simulink model "slexMFSKMultiTargetsExample"  (R2019a)
settings: Solver=FixedStepDiscrete  StartTime=0.0  StopTime=paramMFSKMT.T  RelTol=1e-3  EnableMultiTasking=on
PreLoadFcn:
  | helperslexMFSKMultiTargetsParam
undefined symbols (not defined in the file or in its folder): paramMFSKMT
libraries: phasedenvlib x7, phasedtxrxlib x2, phaseddetectlib x2, dspxfrm3 x2, phasedwavlib x1, dspsolvers x1
CloseFcn:
  | clear paramMFSKMT
Description:
  | FMCW Radar Range Estimation
  | 
  | This model shows how to use a FMCW radar to estimate a target's range.
settings Model: Creator=The MathWorks, Inc.  LastModifiedBy=The MathWorks, Inc.
settings DataIOCC: LimitDataPoints=on  SaveFormat=Array  ReturnWorkspaceOutputs=off
settings OptimizationCC: LifeSpan=inf
settings DebuggingCC: ReadBeforeWriteMsg=DisableAll  WriteAfterWriteMsg=DisableAll  WriteAfterReadMsg=DisableAll  UnderspecifiedInitializationDetection=Classic  MergeDetectMultiDrivingBlocksExec=none  SolverPrmCheckMsg=warning  MultiTaskDSMMsg=none  PregeneratedLibrarySubsystemCodeDiagnostic=none  SFUnexpectedBacktrackingDiag=warning  SFNoUnconditionalDefaultTransitionDiag=warning  SFExecutionAtInitializationDiag=none  ArithmeticOperatorsInVariantConditions=warning
settings HardwareCC: ProdBitPerPointer=32  ProdBitPerSizeT=32  ProdBitPerPtrDiffT=32  ProdLargestAtomicFloat=None  ProdIntDivRoundTo=Undefined  ProdEndianess=Unspecified  ProdWordSize=32  ProdHWDeviceType=32-bit Generic
settings ModelReferenceCC: UpdateModelReferenceTargets=IfOutOfDate  PropagateSignalLabelsOutOfModel=off
settings SFSimCC: SFSimEcho=off  SimUseLocalCustomCode=off
settings RTWCC: RTWUseLocalCustomCode=off
settings CodeAppCC: StateflowObjectComments=on
settings GRTTargetCC: TargetLangStandard=C89/C90 (ANSI)  GeneratePreprocessorConditionals=Disable all
settings ConfigComp: CovMetricSettings=dw  CovHtmlReporting=on  CovSaveCumulativeToWorkspaceVar=on  CovSaveSingleToWorkspaceVar=on  CovExternalEMLEnable=off  CovSFcnEnable=off

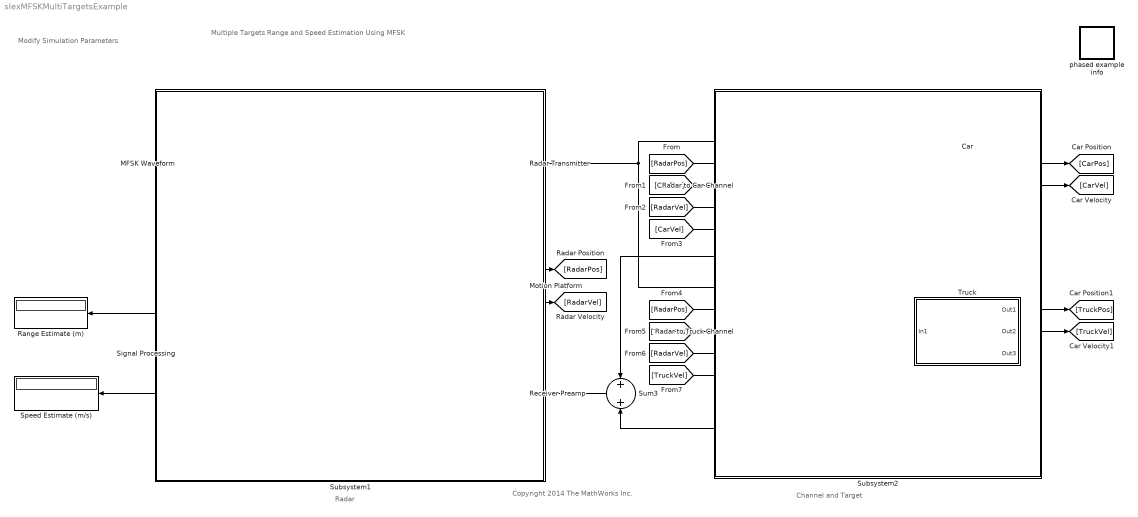
== system slexMFSKMultiTargetsExample ==
  note: Copyright 2014 The MathWorks Inc.
  note: Radar
  note: Channel and Target
  note: Multiple Targets Range and Speed Estimation Using MFSK
  note: Modify Simulation Parameters
  Car : Subsystem
      mask Display:
      | disp('Car')
      | port_label('output',1,'Pos')
      | port_label('output',2,'Vel')
      | port_label('output',3,'Sig')
  MFSK Waveform : phasedwavlib/MFSK Waveform  SampleRate=paramMFSKMT.Fs  SweepBandwidth=paramMFSKMT.bw  StepTime=paramMFSKMT.Tstep  StepsPerSweep=paramMFSKMT.Nstep  FrequencyOffset=paramMFSKMT.Foffset  OutputFormat=Sweeps  NumSamples=100  NumSteps=1  NumSweeps=1  SimulateUsing=Interpreted execution
      settings: SourceProductName=Phased Array System Toolbox  SourceProductBaseCode=AR
  Motion Platform : phasedenvlib/Motion Platform  MotionModel=Velocity  InitialPosition=paramMFSKMT.RadarPos  InitialVelocity=[ 0; 0; 0 ]  VelocitySource=Property  Velocity=paramMFSKMT.RadarVel  AccelerationSource=Property  Acceleration=[0;0;0]  CustomTrajectory=[ 0, 0, 0, 0, 0, 0, 0; 1, 0, 0, 0, 0, 0, 0 ]  ScanMode=None  InitialScanAngle=0  AzimuthSpan=[ -60, 60 ]  AzimuthScanRate=10  InitialOrientationAxes=eye( 3 )  OrientationAxesOutputPort=off  ElapsedTimeSource=Auto  SampleRateFromInputCheckbox=on  SampleRate=1e6  SimulateUsing=Interpreted execution
      settings: SourceProductName=Phased Array System Toolbox  SourceProductBaseCode=AR
  Radar Transmitter : phasedtxrxlib/Transmitter  PeakPower=paramMFSKMT.ppow  Gain=paramMFSKMT.TxGain  LossFactor=0  InUseOutputPort=off  CoherentOnTransmit=on  PhaseNoiseOutputPort=off  SeedSource=Auto  Seed=0  SimulateUsing=Interpreted execution
      settings: SourceProductName=Phased Array System Toolbox  SourceProductBaseCode=AR
  Radar to Car Channel : phasedenvlib/Free Space  PropagationSpeed=paramMFSKMT.C  OperatingFrequency=paramMFSKMT.Fc  TwoWayPropagation=on  SampleRateFromInputCheckbox=on  SampleRate=1e6  MaximumDistanceSource=Property  MaximumDistance=500  MaximumNumInputSamplesSource=Auto  MaximumNumInputSamples=1000  SimulateUsing=Interpreted execution
      settings: SourceProductName=Phased Array System Toolbox  SourceProductBaseCode=AR
  Radar to Truck Channel : phasedenvlib/Free Space  PropagationSpeed=paramMFSKMT.C  OperatingFrequency=paramMFSKMT.Fc  TwoWayPropagation=on  SampleRateFromInputCheckbox=on  SampleRate=1e6  MaximumDistanceSource=Property  MaximumDistance=500  MaximumNumInputSamplesSource=Auto  MaximumNumInputSamples=1000  SimulateUsing=Interpreted execution
      settings: SourceProductName=Phased Array System Toolbox  SourceProductBaseCode=AR
  Range Estimate (m) : Display
  Receiver Preamp : phasedtxrxlib/Receiver Preamp  Gain=paramMFSKMT.RxGain  LossFactor=0  NoiseMethod=Noise temperature  NoiseFigure=paramMFSKMT.NF  ReferenceTemperature=290  SampleRateFromInputCheckbox=on  SampleRate=1e6  NoisePower=0  EnableInputPort=off  PhaseNoiseInputPort=off  SeedSource=Auto  Seed=0  SimulateUsing=Interpreted execution
      settings: SourceProductName=Phased Array System Toolbox  SourceProductBaseCode=AR
  Signal Processing : Subsystem
      mask Display:
      | disp('Signal\nProcessing')
      | port_label('input',1,'Ref')
      | port_label('input',2,'Echo')
      | port_label('output',1,'Range')
      | port_label('output',2,'Speed')
  Speed Estimate (m/s) : Display
  Subsystem1 : Subsystem
  Subsystem2 : Subsystem
  Sum3 : Sum  Inputs=+|+
  Truck : Subsystem
      mask Display:
      | disp('Truck')
      | port_label('output',1,'Pos')
      | port_label('output',2,'Vel')
      | port_label('output',3,'Sig')
  phased example info : Subsystem
      settings: OpenFcn=|
      | modelname = 'slexFMCWExample';
      | helpview(fullfile(matlabroot,'help','phased','helptargets.map'),sprintf('%sExample',modelname));
      | clear modelname;
      mask Display: disp('Info')
  wires:
  MFSK Waveform/1 -> Signal Processing/1(In1), Radar Transmitter/1
  [RadarPos] -> Radar to Car Channel/2
  [CarPos] -> Radar to Car Channel/3
  [RadarVel] -> Radar to Car Channel/4
  [CarVel] -> Radar to Car Channel/5
  Radar Transmitter/1 -> Radar to Truck Channel/1, Radar to Car Channel/1
  Motion Platform/1 -> [RadarPos]
  Motion Platform/2 -> [RadarVel]
  Radar to Car Channel/1 -> Car/1(In1)
  Car/1(Out1) -> [CarPos]
  Car/2(Out2) -> [CarVel]
  Truck/1(Out1) -> [TruckPos]
  Truck/2(Out2) -> [TruckVel]
  Radar to Truck Channel/1 -> Truck/1(In1)
  [RadarPos] -> Radar to Truck Channel/2
  [TruckPos] -> Radar to Truck Channel/3
  [RadarVel] -> Radar to Truck Channel/4
  [TruckVel] -> Radar to Truck Channel/5
  Car/3(Out3) -> Sum3/1
  Sum3/1 -> Receiver Preamp/1
  Truck/3(Out3) -> Sum3/2
  Receiver Preamp/1 -> Signal Processing/2(In2)
  Signal Processing/1(Out1) -> Range Estimate (m)/1
  Signal Processing/2(Out2) -> Speed Estimate (m/s)/1

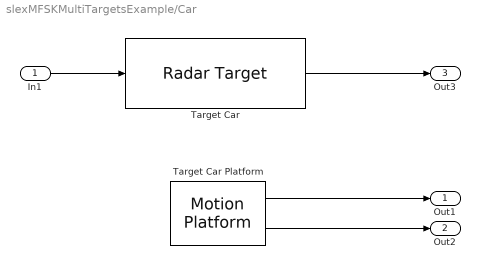
== system slexMFSKMultiTargetsExample/Car ==
  In1 : Inport
  Target Car : phasedenvlib/Radar Target  EnablePolarization=off  Mode=Monostatic  MeanRCSSource=Property  ScatteringMatrixSource=Property  MeanRCS=paramMFSKMT.RCS  ScatteringMatrix=eye( 2 )  Model=Nonfluctuating  PropagationSpeed=paramMFSKMT.C  OperatingFrequency=paramMFSKMT.Fc  SeedSource=Auto  Seed=0  SimulateUsing=Interpreted execution
      settings: SourceProductName=Phased Array System Toolbox  SourceProductBaseCode=AR
  Target Car Platform : phasedenvlib/Motion Platform  MotionModel=Velocity  InitialPosition=paramMFSKMT.CarPos  InitialVelocity=[ 0; 0; 0 ]  VelocitySource=Property  Velocity=paramMFSKMT.CarVel  AccelerationSource=Property  Acceleration=[0;0;0]  CustomTrajectory=[ 0, 0, 0, 0, 0, 0, 0; 1, 0, 0, 0, 0, 0, 0 ]  ScanMode=None  InitialScanAngle=0  AzimuthSpan=[ -60, 60 ]  AzimuthScanRate=10  InitialOrientationAxes=eye( 3 )  OrientationAxesOutputPort=off  ElapsedTimeSource=Auto  SampleRateFromInputCheckbox=on  SampleRate=1e6  SimulateUsing=Interpreted execution
      settings: SourceProductName=Phased Array System Toolbox  SourceProductBaseCode=AR
  Out1 : Outport
  Out2 : Outport  Port=2
  Out3 : Outport  Port=3
  wires:
  Target Car/1 -> Out3/1
  In1/1 -> Target Car/1
  Target Car Platform/1 -> Out1/1
  Target Car Platform/2 -> Out2/1

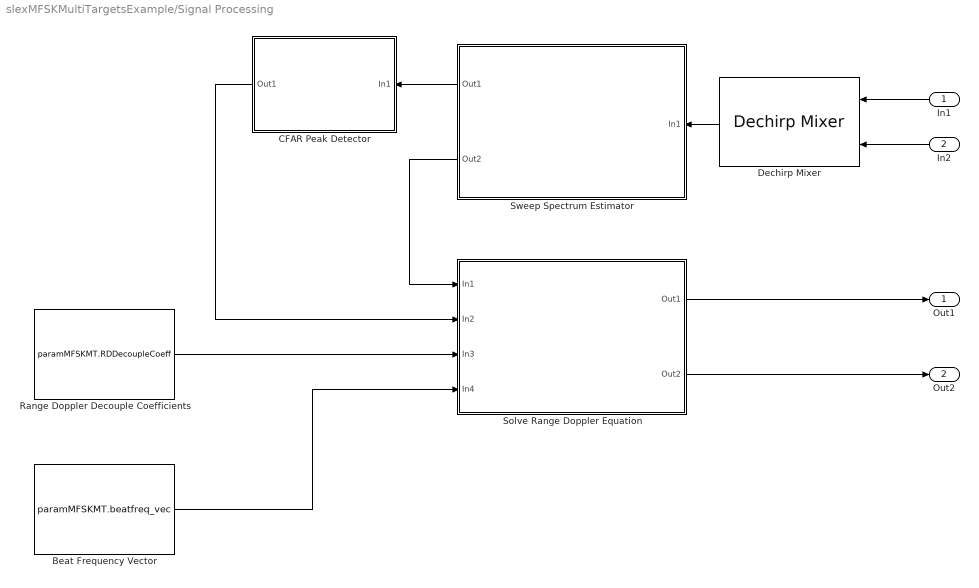
== system slexMFSKMultiTargetsExample/Signal Processing ==
  In1 : Inport
  In2 : Inport  Port=2
  Beat Frequency Vector : Constant  Value=paramMFSKMT.beatfreq_vec  VectorParams1D=off
  CFAR Peak Detector : Subsystem
      mask Display:
      | disp('Peak\nIndex')
      | port_label('output',1,'Idx')
  Dechirp Mixer : phaseddetectlib/Dechirp Mixer
      settings: SourceProductName=Phased Array System Toolbox  SourceProductBaseCode=AR
  Range Doppler Decouple Coefficients : Constant  Value=paramMFSKMT.RDDecoupleCoeff  VectorParams1D=off
  Solve Range Doppler Equation : Subsystem
      mask Display:
      | disp('Range\nDopppler\nSolver\nAX=B')
      | port_label('output',1,'range')
      | port_label('output',2,'speed')
      | port_label('input',2,'Beat Idx')
      | port_label('input',1,'\Delta\Phi_{sweep}','texmode','on')
      | port_label('input',3,'A')
      | port_label('input',4,'freq')
  Sweep Spectrum Estimator : Subsystem
      mask Display:
      | disp('Sweep\nSpectrum')
      | port_label('input',1,'X_d','texmode','on')
      | port_label('output',1,'|F_{sweep}|','texmode','on')
      | port_label('output',2,'\Delta\Phi_{sweep}','texmode','on')
  Out1 : Outport
  Out2 : Outport  Port=2
  wires:
  In2/1 -> Dechirp Mixer/2
  In1/1 -> Dechirp Mixer/1
  Dechirp Mixer/1 -> Sweep Spectrum Estimator/1(In1)
  Sweep Spectrum Estimator/1(Out1) -> CFAR Peak Detector/1(In1)
  Range Doppler Decouple Coefficients/1 -> Solve Range Doppler Equation/3(In3)
  Beat Frequency Vector/1 -> Solve Range Doppler Equation/4(In4)
  Solve Range Doppler Equation/1(Out1) -> Out1/1
  Solve Range Doppler Equation/2(Out2) -> Out2/1
  Sweep Spectrum Estimator/2(Out2) -> Solve Range Doppler Equation/1(In1)
  CFAR Peak Detector/1(Out1) -> Solve Range Doppler Equation/2(In2)

== system slexMFSKMultiTargetsExample/Subsystem1 ==

== system slexMFSKMultiTargetsExample/Subsystem2 ==

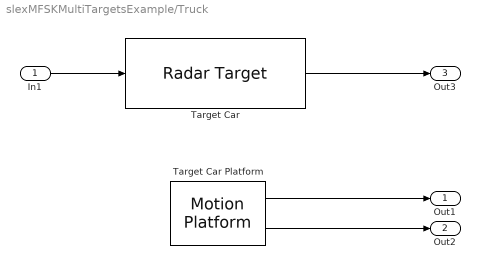
== system slexMFSKMultiTargetsExample/Truck ==
  In1 : Inport
  Target Car : phasedenvlib/Radar Target  EnablePolarization=off  Mode=Monostatic  MeanRCSSource=Property  ScatteringMatrixSource=Property  MeanRCS=paramMFSKMT.TruckRCS  ScatteringMatrix=eye( 2 )  Model=Nonfluctuating  PropagationSpeed=paramMFSKMT.C  OperatingFrequency=paramMFSKMT.Fc  SeedSource=Auto  Seed=0  SimulateUsing=Interpreted execution
      settings: SourceProductName=Phased Array System Toolbox  SourceProductBaseCode=AR
  Target Car Platform : phasedenvlib/Motion Platform  MotionModel=Velocity  InitialPosition=paramMFSKMT.TruckPos  InitialVelocity=[ 0; 0; 0 ]  VelocitySource=Property  Velocity=paramMFSKMT.TruckVel  AccelerationSource=Property  Acceleration=[0;0;0]  CustomTrajectory=[ 0, 0, 0, 0, 0, 0, 0; 1, 0, 0, 0, 0, 0, 0 ]  ScanMode=None  InitialScanAngle=0  AzimuthSpan=[ -60, 60 ]  AzimuthScanRate=10  InitialOrientationAxes=eye( 3 )  OrientationAxesOutputPort=off  ElapsedTimeSource=Auto  SampleRateFromInputCheckbox=on  SampleRate=1e6  SimulateUsing=Interpreted execution
      settings: SourceProductName=Phased Array System Toolbox  SourceProductBaseCode=AR
  Out1 : Outport
  Out2 : Outport  Port=2
  Out3 : Outport  Port=3
  wires:
  Target Car Platform/2 -> Out2/1
  Target Car Platform/1 -> Out1/1
  In1/1 -> Target Car/1
  Target Car/1 -> Out3/1

== system slexMFSKMultiTargetsExample/phased example info ==

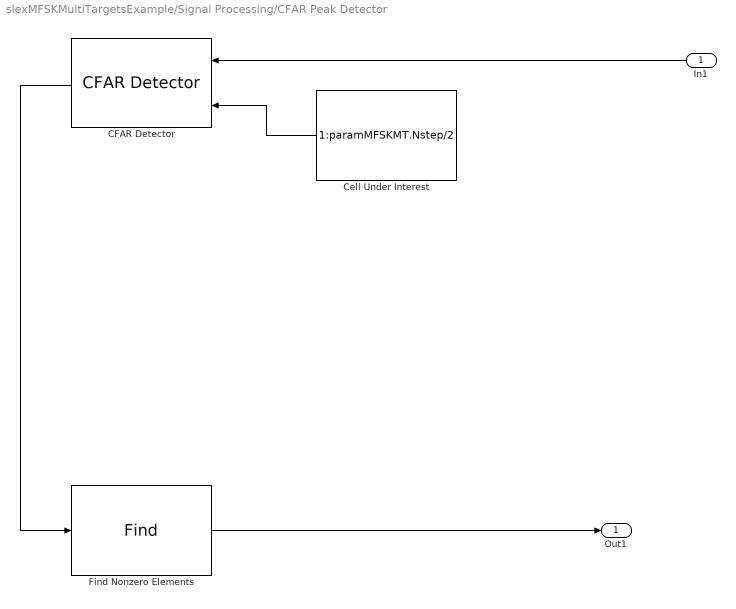
== system slexMFSKMultiTargetsExample/Signal Processing/CFAR Peak Detector ==
  In1 : Inport
  CFAR Detector : phaseddetectlib/CFAR Detector  Method=CA  Rank=1  NumGuardCells=2  NumTrainingCells=8  ThresholdFactor=Auto  ProbabilityFalseAlarm=0.001  CustomThresholdFactor=1  OutputFormat=CUT result  ThresholdOutputPort=off  NoisePowerOutputPort=off  NumDetectionsSource=Auto  NumDetections=1  SimulateUsing=Interpreted execution
      settings: SourceProductName=Phased Array System Toolbox  SourceProductBaseCode=AR
  Cell Under Interest : Constant  Value=1:paramMFSKMT.Nstep/2
  Find Nonzero Elements : Find  NumberOfInputDimensions=3
  Out1 : Outport
  wires:
  Cell Under Interest/1 -> CFAR Detector/2
  CFAR Detector/1 -> Find Nonzero Elements/1
  In1/1 -> CFAR Detector/1
  Find Nonzero Elements/1 -> Out1/1

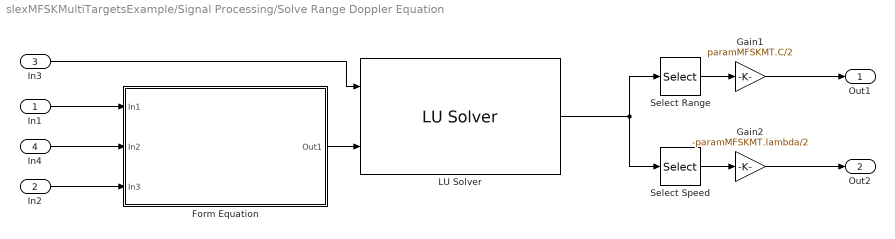
== system slexMFSKMultiTargetsExample/Signal Processing/Solve Range Doppler Equation ==
  In1 : Inport
  In2 : Inport  Port=2
  In3 : Inport  Port=3
  In4 : Inport  Port=4
  Form Equation : Subsystem
      mask Display:
      | disp('Coupled\nRange Doppler')
      | port_label('input',1,'\Delta\Phi','texmode','on')
      | port_label('input',2,'freq')
      | port_label('input',3,'Idx')
      | port_label('output',1,'B')
  Gain1 : Gain  Gain=paramMFSKMT.C/2
  Gain2 : Gain  Gain=-paramMFSKMT.lambda/2
  LU Solver : dspsolvers/LU Solver
      settings: SourceProductName=DSP System Toolbox  SourceProductBaseCode=DS
  Select Range : Selector  NumberOfDimensions=2  InputPortWidth=3  IndexOptions=Index vector (dialog),Select all  Indices=1,1  OutputSizes=1,1
  Select Speed : Selector  NumberOfDimensions=2  InputPortWidth=3  IndexOptions=Index vector (dialog),Select all  Indices=2,1  OutputSizes=1,1
  Out1 : Outport
  Out2 : Outport  Port=2
  wires:
  In3/1 -> LU Solver/1
  Select Range/1 -> Gain1/1
  LU Solver/1 -> Select Speed/1, Select Range/1
  Select Speed/1 -> Gain2/1
  Gain1/1 -> Out1/1
  Gain2/1 -> Out2/1
  In4/1 -> Form Equation/2(In2)
  Form Equation/1(Out1) -> LU Solver/2
  In1/1 -> Form Equation/1(In1)
  In2/1 -> Form Equation/3(In3)

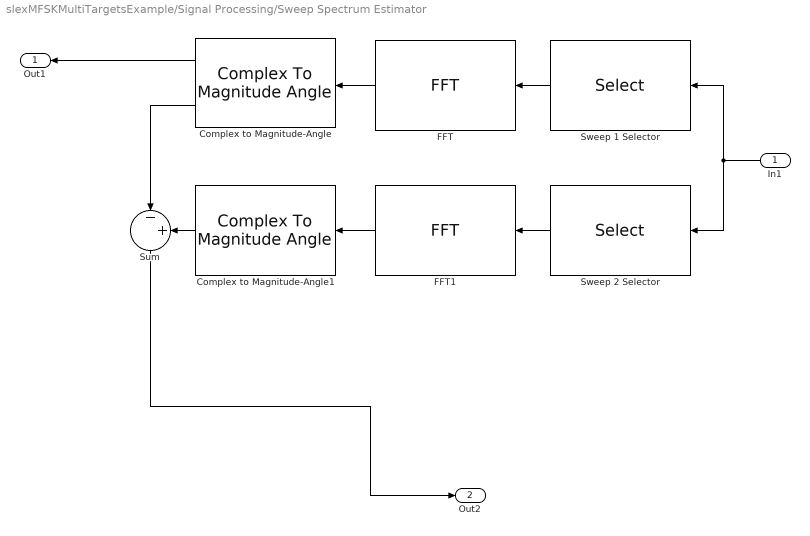
== system slexMFSKMultiTargetsExample/Signal Processing/Sweep Spectrum Estimator ==
  In1 : Inport
  Complex to Magnitude-Angle : ComplexToMagnitudeAngle
  Complex to Magnitude-Angle1 : ComplexToMagnitudeAngle  Output=Angle
  FFT : dspxfrm3/FFT  FFTImplementation=Auto  CompMethod=Table lookup  TableOpt=NEW  TableOptActive=Speed  BitRevOrder=off  Normalize=off  InheritFFTLength=on  FFTLength=64  WrapInput=on  roundingMode=Floor  overflowMode=off  firstCoeffDataTypeStr=Inherit: Same word length as input  firstCoeffLastDataTypeStr=Inherit: Same word length as input  outputMin=[]  outputMax=[]
  FFT1 : dspxfrm3/FFT  FFTImplementation=Auto  CompMethod=Table lookup  TableOpt=NEW  TableOptActive=Speed  BitRevOrder=off  Normalize=off  InheritFFTLength=on  FFTLength=64  WrapInput=on  roundingMode=Floor  overflowMode=off  firstCoeffDataTypeStr=Inherit: Same word length as input  firstCoeffLastDataTypeStr=Inherit: Same word length as input  outputMin=[]  outputMax=[]
  Sum : Sum  Inputs=|-+
  Sweep 1 Selector : Selector  NumberOfDimensions=2  InputPortWidth=3  IndexOptions=Index vector (dialog),Index vector (dialog)  Indices=(1:2:paramMFSKMT.Nstep)*paramMFSKMT.Nsampperstep,1  OutputSizes=1,1
  Sweep 2 Selector : Selector  NumberOfDimensions=2  InputPortWidth=3  IndexOptions=Index vector (dialog),Index vector (dialog)  Indices=(2:2:paramMFSKMT.Nstep)*paramMFSKMT.Nsampperstep,1  OutputSizes=1,1
  Out1 : Outport
  Out2 : Outport  Port=2
  wires:
  In1/1 -> Sweep 1 Selector/1, Sweep 2 Selector/1
  Sweep 1 Selector/1 -> FFT/1
  Sweep 2 Selector/1 -> FFT1/1
  FFT1/1 -> Complex to Magnitude-Angle1/1
  FFT/1 -> Complex to Magnitude-Angle/1
  Complex to Magnitude-Angle/1 -> Out1/1
  Complex to Magnitude-Angle1/1 -> Sum/2
  Complex to Magnitude-Angle/2 -> Sum/1
  Sum/1 -> Out2/1

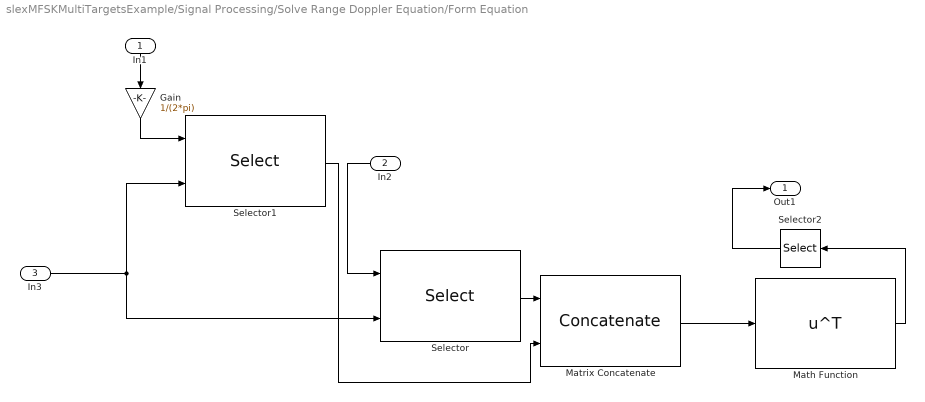
== system slexMFSKMultiTargetsExample/Signal Processing/Solve Range Doppler Equation/Form Equation ==
  In1 : Inport
  In2 : Inport  Port=2
  In3 : Inport  Port=3
  Gain : Gain  Gain=1/(2*pi)
  Math Function : Math  Operator=transpose  SaturateOnIntegerOverflow=on
  Matrix Concatenate : Concatenate  Mode=Multidimensional array  ConcatenateDimension=2
  Selector : Selector  NumberOfDimensions=2  InputPortWidth=3  IndexOptions=Index vector (port),Index vector (dialog)  Indices=[1 3],1  OutputSizes=1,1
  Selector1 : Selector  NumberOfDimensions=2  InputPortWidth=3  IndexOptions=Index vector (port),Index vector (dialog)  Indices=[1 3],1  OutputSizes=1,1
  Selector2 : Selector  NumberOfDimensions=2  InputPortWidth=3  IndexOptions=Index vector (dialog),Index vector (dialog)  Indices=[1 2],[1 2]  OutputSizes=1,1
  Out1 : Outport
  wires:
  In2/1 -> Selector/1
  In3/1 -> Selector1/2, Selector/2
  In1/1 -> Gain/1
  Selector/1 -> Matrix Concatenate/1
  Selector1/1 -> Matrix Concatenate/2
  Matrix Concatenate/1 -> Math Function/1
  Math Function/1 -> Selector2/1
  Selector2/1 -> Out1/1
  Gain/1 -> Selector1/1
